simulink model "req2"  (R2019a)
settings: Solver=FixedStepAuto  StartTime=0.0  StopTime=100  RelTol=1e-3
libraries: sldvlib x1
settings Model: Creator=e40014285  LastModifiedBy=e40014285

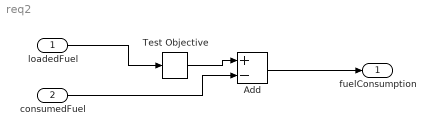
== system req2 ==
  loadedFuel : Inport  OutDataTypeStr=double
  consumedFuel : Inport  Port=2  OutDataTypeStr=double
  Add : Sum  Inputs=+-
  Test Objective : sldvlib/Objectives and Constraints/Test Objective  enabled=on  customAVTBlockType=Test Objective  intervals={0,1}  dispValues=on  outEnabled=on
      settings: AttributesFormatString=%<intervals>  SourceProductName=Simulink  SourceProductBaseCode=SL
  fuelConsumption : Outport  OutDataTypeStr=double
  wires:
  consumedFuel/1 -> Add/2
  loadedFuel/1 -> Test Objective/1
  Add/1 -> fuelConsumption/1
  Test Objective/1 -> Add/1
